simulink model "planRoute_ros"  (R2024a)
settings: Solver=FixedStepAuto  StartTime=0.0  StopTime=10.0  RelTol=1e-3
InitFcn:
  | % Make sure server is running
  | svrMdlName = 'routePlanServer';
  | load_system(svrMdlName);
  | set_param(svrMdlName,'SimulationCommand','Start');
  | pause(1);
StopFcn:
  | % Make sure server is running
  | svrMdlName = 'routePlanServer';
  | load_system(svrMdlName);
  | set_param(svrMdlName,'SimulationCommand','Stop');
model workspace (MAT data in the model file):
  SL_ROS_VariableLengthArrays_MaxSizes.CommonInfo.ArrayTruncateAction = 'EmitWarning'
  SL_ROS_VariableLengthArrays_MaxSizes.MsgTypeMap = containers.Map
  SL_ROS_VariableLengthArrays_MaxSizes.MsgTypeMap.serialization.keys = {'std_msgs/Float64MultiArray', 'std_msgs/Int8MultiArray'}
  SL_ROS_VariableLengthArrays_MaxSizes.MsgTypeMap.serialization.values{1}.PropertyName = 'data'
  SL_ROS_VariableLengthArrays_MaxSizes.MsgTypeMap.serialization.values{1}.DataType = 'double'
  SL_ROS_VariableLengthArrays_MaxSizes.MsgTypeMap.serialization.values{1}.MaxLength = 1500000
  SL_ROS_VariableLengthArrays_MaxSizes.MsgTypeMap.serialization.values{2}.PropertyName = 'data'
  SL_ROS_VariableLengthArrays_MaxSizes.MsgTypeMap.serialization.values{2}.DataType = 'int8'
  SL_ROS_VariableLengthArrays_MaxSizes.MsgTypeMap.serialization.values{2}.MaxLength = 1500000
  SL_ROS_VariableLengthArrays_MaxSizes.MsgTypeMap.serialization.uniformity = 0
  SL_ROS_VariableLengthArrays_MaxSizes.MsgTypeMap.serialization.keyType = 'char'
  SL_ROS_VariableLengthArrays_MaxSizes.MsgTypeMap.serialization.valueType = 'any'
undefined symbols (not defined in the file): goal, gridLoc, pathBus_struct, res, start, tuneableTerrainAwareParams, worldMat
libraries: roshelperlib x6, ros2lib x2
settings Model: Creator=cstabile  LastModifiedBy=cstabile
settings OptimizationCC: EnhancedBackFolding=on  PassReuseOutputArgsAs=Individual arguments  ZeroExternalMemoryAtStartup=off  ZeroInternalMemoryAtStartup=off  MaxStackSize=64  OptimizeBlockOrder=speed  DifferentSizesBufferReuse=on  OptimizationCustomize=off  EfficientTunableParamExpr=on
settings DebuggingCC: ParameterTunabilityLossMsg=error
settings SFSimCC: MATLABDynamicMemAlloc=off
settings RTWCC: Description=Embedded Coder  SystemTargetFile=ert.tlc  HardwareBoard=Robot Operating System 2 (ROS 2)  TLCOptions="-aInlineSetEventsForThisBaseRateFcn=TLC_FALSE -aSuppressMultiTaskScheduler=TLC_FALSE  -aRateBasedStepFcn=0"  TemplateMakefile=ert_default_tmf  Toolchain=Colcon Tools  TargetLang=C++
settings CodeAppCC: ForceParamTrailComments=on  IgnoreCustomStorageClasses=off  OperatorAnnotations=on  SimulinkDataObjDesc=on  SFDataObjDesc=on  InsertBlockDesc=on
settings ERTTargetCC: CodeInterfacePackaging=C++ class  RootIOFormat=Structure reference

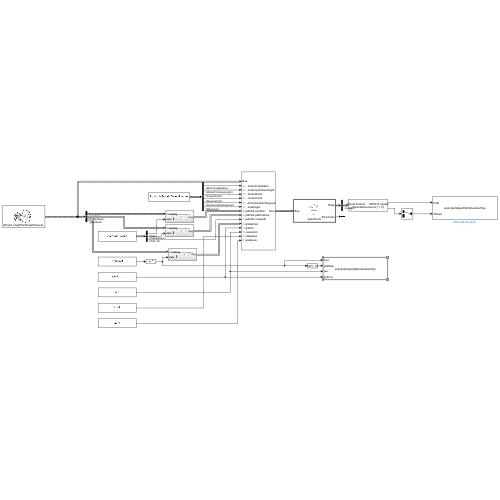
[thumbnail: Simulink's stored preview of the top-level diagram]
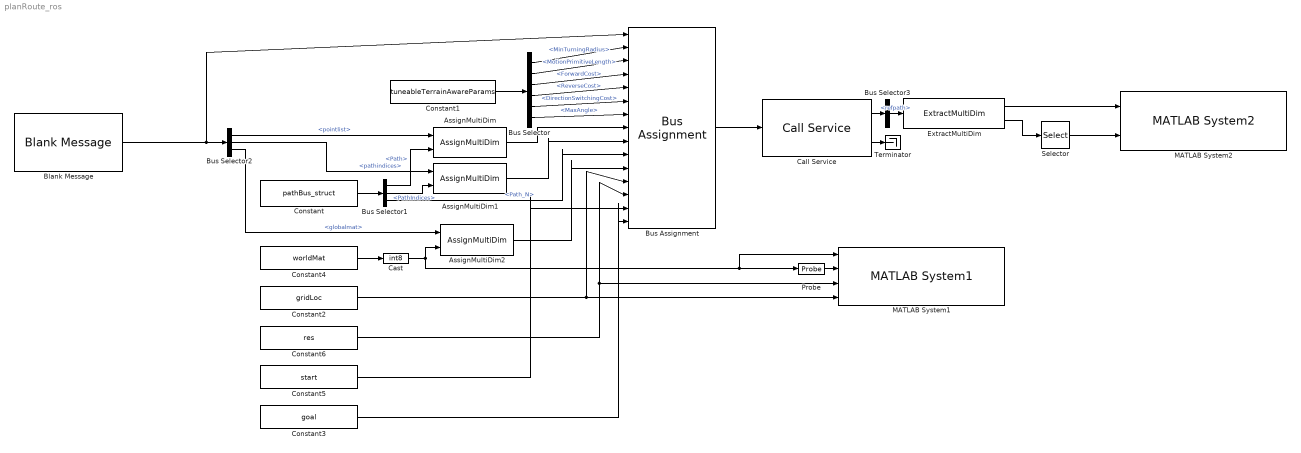
== system planRoute_ros ==
  AssignMultiDim : roshelperlib/AssignMultiDim  SystemSampleTime=-1  VariantActivationTime=update diagram  AllowFlexibleInterface=on  Latency=0  AutoFrameSizeCalculation=off
  AssignMultiDim1 : roshelperlib/AssignMultiDim  SystemSampleTime=-1  VariantActivationTime=update diagram  AllowFlexibleInterface=on  Latency=0  AutoFrameSizeCalculation=off
  AssignMultiDim2 : roshelperlib/AssignMultiDim  SystemSampleTime=-1  VariantActivationTime=update diagram  AllowFlexibleInterface=on  Latency=0  AutoFrameSizeCalculation=off
  Blank Message : ros2lib/Blank Message  messageClass=Service Request  entityType=offroad_msg/PlanRoute  messageType=offroad_msg/PlanRouteRequest  SampleTime=inf
  Bus Assignment : BusAssignment  AssignedSignals=tuneableterrainawareparams.minturningradius,tuneableterrainawareparams.motionprimitivelength,tuneableterrainawareparams.forwardcost,tuneableterrainawareparams.reversecost,tuneableterrainawareparams.directionswitchingcost,tuneableterrainawareparams.maxangle,pathlist.pointlist,pathlist.pathindices,pathlist.numpath,globalmat,gridloc,resolution,startpose,goalpose
  Bus Selector : BusSelector  OutputSignals=MinTurningRadius,MotionPrimitiveLength,ForwardCost,ReverseCost,DirectionSwitchingCost,MaxAngle
  Bus Selector1 : BusSelector  OutputSignals=Path,PathIndices,Path_N
  Bus Selector2 : BusSelector  OutputSignals=pathlist.pointlist,pathlist.pathindices,globalmat
  Bus Selector3 : BusSelector  OutputSignals=refpath
  Call Service : ros2lib/Call Service  topicSource=Specify your own  service=/planRoute  serviceType=offroad_msg/PlanRoute  connectionTimeout=5  ShowErrorCodeOutput=on  legacyBusStruct=off  QOSHistory=Keep last  QOSDepth=1  QOSReliability=Reliable  QOSDurability=Volatile  QOSDeadline=Inf  QOSLifespan=Inf  QOSLiveliness=Automatic  QOSLeaseDuration=Inf  QOSAvoidROSNamespaceConventions=off
  Cast : DataTypeConversion  OutDataTypeStr=int8  SaturateOnIntegerOverflow=off  RndMeth=Floor
  Constant : Constant  Value=pathBus_struct  VectorParams1D=off  OutDataTypeStr=Bus: pathList_fixed_bus  SampleTime=-1
  Constant1 : Constant  Value=tuneableTerrainAwareParams  OutDataTypeStr=Bus: fsp_tunable_bus
  Constant2 : Constant  Value=gridLoc
  Constant3 : Constant  Value=goal
  Constant4 : Constant  Value=worldMat
  Constant5 : Constant  Value=start
  Constant6 : Constant  Value=res
  ExtractMultiDim : roshelperlib/ExtractMultiDim  userDataType=double  dims=[1e4 3]  isVarsize=on  varsizeDims=[1 0]  returnFixedTF=on
  MATLAB System1 : roshelperlib/MATLAB System1  MapType=SDF  DisplayVisual=on  SimulateUsing=Interpreted execution
  MATLAB System2 : roshelperlib/MATLAB System2  VisualizationParameters={'k-'}  PlotType=Line  DisplayVisual=on  SimulateUsing=Interpreted execution
  Probe : Probe  ProbeWidth=off  ProbeSampleTime=off  ProbeComplexSignal=off  ProbeSignalDimensions=on
  Selector : Selector  InputPortWidth=2  IndexOptions=Index vector (dialog)  Indices=1  OutputSizes=1
  Terminator : Terminator
  wires:
  Blank Message/1 -> Bus Assignment/1, Bus Selector2/1
  Constant1/1 -> Bus Selector/1
  Bus Selector/6 -> Bus Assignment/7  "<MaxAngle>"
  Bus Selector/5 -> Bus Assignment/6  "<DirectionSwitchingCost>"
  Bus Selector/4 -> Bus Assignment/5  "<ReverseCost>"
  Bus Selector/3 -> Bus Assignment/4  "<ForwardCost>"
  Bus Selector/2 -> Bus Assignment/3  "<MotionPrimitiveLength>"
  Bus Selector/1 -> Bus Assignment/2  "<MinTurningRadius>"
  Constant/1 -> Bus Selector1/1
  Bus Selector2/1 -> AssignMultiDim/1  "<pointlist>"
  Bus Selector2/2 -> AssignMultiDim1/1  "<pathindices>"
  Bus Selector1/1 -> AssignMultiDim/2  "<Path>"
  Bus Selector1/2 -> AssignMultiDim1/2  "<PathIndices>"
  AssignMultiDim/1 -> Bus Assignment/8
  AssignMultiDim1/1 -> Bus Assignment/9
  Bus Selector1/3 -> Bus Assignment/10  "<Path_N>"
  Bus Selector2/3 -> AssignMultiDim2/1  "<globalmat>"
  Constant4/1 -> Cast/1
  Cast/1 -> AssignMultiDim2/2, MATLAB System1/1, Probe/1
  AssignMultiDim2/1 -> Bus Assignment/11
  Constant2/1 -> Bus Assignment/12, MATLAB System1/4
  Constant6/1 -> Bus Assignment/13, MATLAB System1/3
  Constant5/1 -> Bus Assignment/14
  Constant3/1 -> Bus Assignment/15
  Bus Assignment/1 -> Call Service/1
  Call Service/1 -> Bus Selector3/1
  Call Service/2 -> Terminator/1
  Bus Selector3/1 -> ExtractMultiDim/1  "<refpath>"
  Probe/1 -> MATLAB System1/2
  ExtractMultiDim/1 -> MATLAB System2/1
  ExtractMultiDim/2 -> Selector/1
  Selector/1 -> MATLAB System2/2
